simulink model "gm_sampleModel1510_2_sub"  (R2023a)
settings: Solver=VariableStepAuto  StartTime=0.0  StopTime=10.0  RelTol=1e-3
libraries: simulink x3
settings Model: Creator=user1  LastModifiedBy=user1
settings OptimizationCC: BlockReduction=off  ConditionallyExecuteInputs=off
settings DebuggingCC: InheritedTsInSrcMsg=none

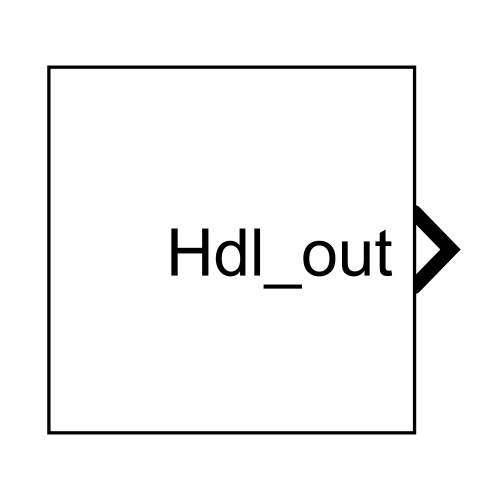
[thumbnail: Simulink's stored preview of the top-level diagram]
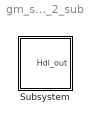
== system gm_sampleModel1510_2_sub ==
  Subsystem : Subsystem

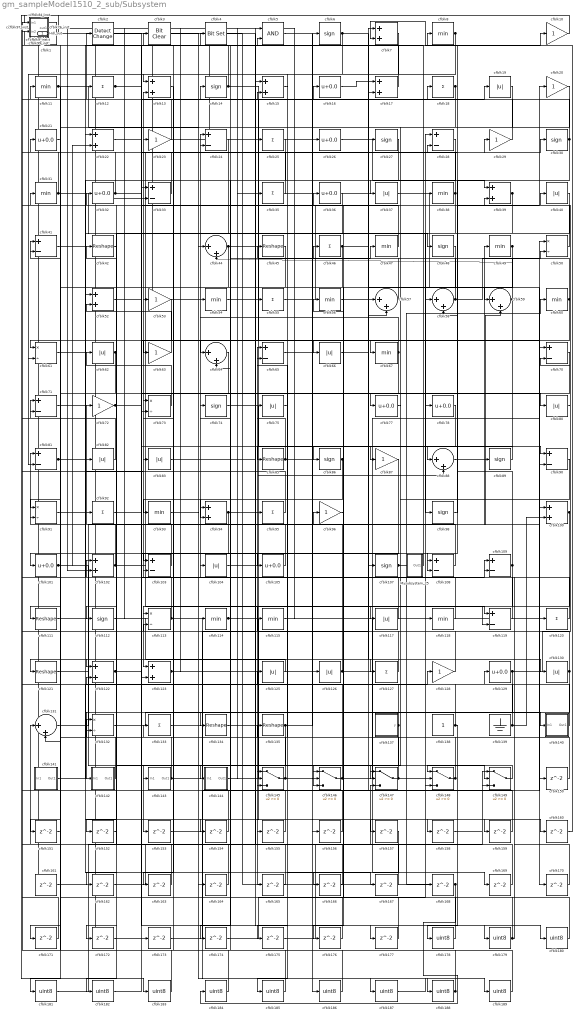
== system gm_sampleModel1510_2_sub/Subsystem ==
  Mysubsystem_25 : Subsystem
  cfblk1 : RelationalOperator  Operator=<=  OutDataTypeStr=boolean  InputSameDT=off
  cfblk{10,20,23,29,53,63,72,87,96,128} (10 alike) : Gain  OutDataTypeStr=uint8
  cfblk{7,13,15,17,22,39,52,94,100,102,122..123} (12 alike) : Sum  OutDataTypeStr=uint8
  cfblk{16,21,26,32,36,77..78,101,105,129} (10 alike) : Bias  Bias=0.0  SaturateOnIntegerOverflow=off
  cfblk{24,28,33,41,65,70..71,81,90,103,108..109,119} (13 alike) : Sum  Inputs=+-  OutDataTypeStr=uint8
  cfblk{19,37,40,62,66,75,80,82..83,104,117,125..126,130} (14 alike) : Abs  OutDataTypeStr=uint8  SaturateOnIntegerOverflow=off
  cfblk106_inst : Subsystem
  cfblk{6,14,27,30,48,74,86,89,98,107,112} (11 alike) : Signum
  cfblk{8,11,31,38,47,49,54,56,60,67,93,114..115,118} (14 alike) : MinMax  OutDataTypeStr=uint8
  cfblk110_inst : Subsystem
  cfblk{42,45,85,111,121,134..135} (7 alike) : Reshape
  cfblk{50,61,73,91,113,132} (6 alike) : Product  Inputs=*/  OutDataTypeStr=uint8  RndMeth=Zero  SaturateOnIntegerOverflow=on
  cfblk116_inst : Subsystem
  cfblk{12,18,25,35,46,55,92,95,120,127,133} (11 alike) : Sum  Inputs=+  OutDataTypeStr=uint8
  cfblk124_inst : Subsystem
  cfblk{44,57..59,64,88,131} (7 alike) : Sum  Inputs=|++  OutDataTypeStr=uint8
  cfblk137 : Subsystem  mask(Counter Free-Running){NumBits=double(16), tsamp=double(-1)}
      mask prompts: NumBits "Simulink:masks:NumberOfBits_MP"; tsamp "Simulink:masks:SampleTime_MP"
      mask help: Simulink:masks:CounterFreeRunning_MD
  cfblk138 : Constant  OutDataTypeStr=uint8  SampleTime=-1
  cfblk139 : Ground
  cfblk140 : Subsystem
  cfblk141 : Subsystem
  cfblk142 : Subsystem
  cfblk143 : Subsystem
  cfblk144 : Subsystem
  cfblk{145..149} (5 alike) : Switch  OutDataTypeStr=uint8  SaturateOnIntegerOverflow=off  InputSameDT=off
  cfblk{150..177} (28 alike) : Delay  SampleTime=1
  cfblk{178..189} (12 alike) : DataTypeConversion  OutDataTypeStr=uint8  SaturateOnIntegerOverflow=off  RndMeth=Floor
  cfblk2 : simulink/Logic and Bit Operations/Detect Change  vinit=0  OutDataTypeStr=uint8
      settings: LibrarySourceBlock=|
      | hdlsllib/Logic and Bit
      | Operations/Detect
      | Change
  cfblk3 : simulink/Logic and Bit Operations/Bit Clear  iBit=0
      settings: LibrarySourceBlock=|
      | hdlsllib/Logic and Bit
      | Operations/Bit Clear
  cfblk34_inst : Subsystem
  cfblk4 : simulink/Logic and Bit Operations/Bit Set  iBit=0
      settings: LibrarySourceBlock=|
      | hdlsllib/Logic and Bit
      | Operations/Bit Set
  cfblk43_inst : Subsystem
  cfblk5 : Logic  AllPortsSameDT=off  OutDataTypeStr=boolean
  cfblk51_inst : Subsystem
  cfblk68_inst : Subsystem
  cfblk69_inst : Subsystem
  cfblk76_inst : Subsystem
  cfblk84_inst : Subsystem
  cfblk97_inst : Subsystem
  cfblk99_inst : Subsystem
  cfblk9_inst : Subsystem
  Hdl_out : Outport  OutDataTypeStr=uint8  SampleTime=1
  wires:
  Mysubsystem_25/1(Out1) -> cfblk51_inst/2(in2)
  cfblk1/1 -> cfblk183/1
  cfblk10/1 -> cfblk69_inst/1(in1)
  cfblk100/1 -> cfblk24/1, cfblk123/1
  cfblk101/1 -> cfblk22/2, cfblk149/2
  cfblk102/1 -> cfblk119/1, cfblk72/1, cfblk29/1
  cfblk103/1 -> cfblk81/1
  cfblk104/1 -> cfblk30/1
  cfblk105/1 -> cfblk92/1
  cfblk106_inst/1(out1) -> cfblk118/1
  cfblk107/1 -> cfblk168/1, cfblk60/1
  cfblk108/1 -> cfblk42/1
  cfblk109/1 -> cfblk14/1, cfblk165/1
  cfblk11/1 -> cfblk44/1, cfblk111/1
  cfblk110_inst/1(out1) -> cfblk126/1
  cfblk111/1 -> cfblk50/1
  cfblk112/1 -> cfblk156/1
  cfblk113/1 -> cfblk68_inst/1(in1), cfblk52/2, cfblk167/1
  cfblk114/1 -> cfblk158/1, cfblk18/1
  cfblk115/1 -> cfblk160/1
  cfblk116_inst/1(out1) -> cfblk26/1, cfblk173/1, cfblk114/1
  cfblk117/1 -> cfblk41/1
  cfblk118/1 -> cfblk52/1
  cfblk119/1 -> cfblk13/2
  cfblk12/1 -> cfblk77/1, cfblk108/2
  cfblk120/1 -> cfblk104/1
  cfblk121/1 -> cfblk59/2
  cfblk122/1 -> cfblk24/2, cfblk109/1
  cfblk123/1 -> cfblk88/2, cfblk47/1
  cfblk124_inst/1(out1) -> cfblk33/2
  cfblk125/1 -> cfblk121/1
  cfblk126/1 -> cfblk53/1, cfblk169/1, cfblk11/1
  cfblk127/1 -> cfblk65/1
  cfblk128/1 -> cfblk115/1
  cfblk129/1 -> cfblk70/2, cfblk142/1(In1)
  cfblk13/1 -> cfblk103/1
  cfblk130/1 -> cfblk145/3, cfblk106_inst/2(in2)
  cfblk131/1 -> cfblk49/1
  cfblk132/1 -> cfblk140/1(In1)
  cfblk133/1 -> cfblk188/1
  cfblk134/1 -> cfblk57/1
  cfblk135/1 -> cfblk6/1, cfblk153/1, cfblk152/1
  cfblk137/1(y) -> cfblk146/3, cfblk73/1
  cfblk138/1 -> cfblk178/1, cfblk23/1
  cfblk139/1 -> cfblk125/1, cfblk100/2
  cfblk14/1 -> cfblk110_inst/1(in1), cfblk170/1
  cfblk140/1(Out1) -> cfblk71/1
  cfblk141/1(Out1) -> cfblk128/1
  cfblk142/1(Out1) -> cfblk106_inst/1(in1)
  cfblk143/1(Out1) -> cfblk146/1, cfblk116_inst/2(in2), cfblk35/1
  cfblk144/1(Out1) -> cfblk17/2
  cfblk145/1 -> cfblk103/2, cfblk159/1
  cfblk146/1 -> cfblk70/1, cfblk62/1, cfblk124_inst/2(in2)
  cfblk147/1 -> cfblk96/1, cfblk144/1(In1)
  cfblk148/1 -> cfblk82/1, cfblk135/1
  cfblk149/1 -> cfblk148/1
  cfblk15/1 -> cfblk145/1
  cfblk150/1 -> cfblk65/2
  cfblk151/1 -> cfblk91/2
  cfblk152/1 -> cfblk102/1
  cfblk153/1 -> cfblk90/2
  cfblk154/1 -> cfblk41/2
  cfblk155/1 -> cfblk97_inst/2(in2)
  cfblk156/1 -> cfblk132/1
  cfblk157/1 -> cfblk185/1
  cfblk158/1 -> cfblk149/3
  cfblk159/1 -> cfblk71/2
  cfblk16/1 -> cfblk17/1
  cfblk160/1 -> cfblk7/2
  cfblk161/1 -> cfblk28/1
  cfblk162/1 -> cfblk149/1
  cfblk163/1 -> cfblk69_inst/2(in2)
  cfblk164/1 -> cfblk99_inst/2(in2)
  cfblk165/1 -> cfblk122/2
  cfblk166/1 -> cfblk131/1
  cfblk167/1 -> cfblk147/3
  cfblk168/1 -> cfblk184/1, Hdl_out/1
  cfblk169/1 -> cfblk110_inst/2(in2)
  cfblk17/1 -> cfblk43_inst/1(in1)
  cfblk170/1 -> cfblk109/2
  cfblk171/1 -> cfblk34_inst/2(in2)
  cfblk172/1 -> cfblk39/2
  cfblk173/1 -> cfblk57/2
  cfblk174/1 -> cfblk148/3
  cfblk175/1 -> cfblk58/1
  cfblk176/1 -> cfblk64/2
  cfblk177/1 -> cfblk31/1
  cfblk178/1 -> cfblk4/1
  cfblk179/1 -> cfblk129/1, cfblk113/2
  cfblk18/1 -> cfblk15/2, cfblk67/1
  cfblk180/1 -> cfblk36/1
  cfblk181/1 -> cfblk5/1
  cfblk182/1 -> cfblk5/2
  cfblk183/1 -> cfblk21/1
  cfblk184/1 -> cfblk1/1
  cfblk185/1 -> cfblk1/2
  cfblk186/1 -> cfblk3/1
  cfblk187/1 -> cfblk189/1
  cfblk188/1 -> cfblk97_inst/1(in1), cfblk9_inst/2(in2), cfblk74/1
  cfblk189/1 -> cfblk133/1
  cfblk19/1 -> cfblk147/2
  cfblk2/1 -> cfblk90/1
  cfblk20/1 -> cfblk151/1
  cfblk21/1 -> cfblk91/1
  cfblk22/1 -> cfblk19/1
  cfblk23/1 -> cfblk9_inst/1(in1)
  cfblk24/1 -> cfblk63/1
  cfblk25/1 -> cfblk134/1
  cfblk26/1 -> cfblk39/1
  cfblk27/1 -> cfblk132/2
  cfblk28/1 -> cfblk37/1
  cfblk29/1 -> cfblk2/1
  cfblk3/1 -> cfblk187/1
  cfblk30/1 -> cfblk88/1, cfblk84_inst/1(in1)
  cfblk31/1 -> cfblk78/1, cfblk76_inst/2(in2)
  cfblk32/1 -> cfblk66/1, cfblk124_inst/1(in1)
  cfblk33/1 -> cfblk76_inst/1(in1)
  cfblk34_inst/1(out1) -> cfblk12/1
  cfblk35/1 -> cfblk116_inst/1(in1)
  cfblk36/1 -> cfblk162/1
  cfblk37/1 -> cfblk100/1
  cfblk38/1 -> cfblk64/1, cfblk15/1
  cfblk39/1 -> cfblk146/2, cfblk93/1
  cfblk4/1 -> cfblk179/1
  cfblk40/1 -> cfblk145/2
  cfblk41/1 -> cfblk48/1
  cfblk42/1 -> cfblk182/1
  cfblk43_inst/1(out1) -> cfblk161/1
  cfblk44/1 -> cfblk94/2, cfblk123/2, cfblk107/1
  cfblk45/1 -> cfblk94/1
  cfblk46/1 -> cfblk73/2, cfblk10/1
  cfblk47/1 -> cfblk68_inst/2(in2)
  cfblk48/1 -> cfblk101/1
  cfblk49/1 -> cfblk58/2, cfblk176/1
  cfblk5/1 -> cfblk180/1
  cfblk50/1 -> cfblk8/1
  cfblk51_inst/1(out1) -> cfblk38/1
  cfblk52/1 -> cfblk80/1
  cfblk53/1 -> cfblk61/1
  cfblk54/1 -> cfblk98/1
  cfblk55/1 -> cfblk20/1
  cfblk56/1 -> cfblk59/1
  cfblk57/1 -> cfblk51_inst/1(in1)
  cfblk58/1 -> cfblk50/2, cfblk46/1
  cfblk59/1 -> cfblk86/1, cfblk45/1, cfblk44/2
  cfblk6/1 -> cfblk13/1, cfblk119/2
  cfblk60/1 -> cfblk84_inst/2(in2), cfblk108/1, cfblk113/1
  cfblk61/1 -> cfblk166/1
  cfblk62/1 -> cfblk122/1, cfblk171/1
  cfblk63/1 -> cfblk32/1
  cfblk64/1 -> cfblk131/2
  cfblk65/1 -> cfblk186/1
  cfblk66/1 -> cfblk130/1
  cfblk67/1 -> cfblk163/1, cfblk54/1
  cfblk68_inst/1(out1) -> cfblk120/1
  cfblk69_inst/1(out1) -> cfblk27/1
  cfblk7/1 -> cfblk85/1
  cfblk70/1 -> cfblk172/1
  cfblk71/1 -> cfblk7/1
  cfblk72/1 -> cfblk33/1, cfblk16/1
  cfblk73/1 -> cfblk22/1
  cfblk74/1 -> cfblk150/1
  cfblk75/1 -> cfblk175/1
  cfblk76_inst/1(out1) -> cfblk141/1(In1)
  cfblk77/1 -> cfblk147/1
  cfblk78/1 -> cfblk105/1
  cfblk8/1 -> cfblk81/2, cfblk61/2
  cfblk80/1 -> cfblk40/1
  cfblk81/1 -> cfblk155/1, cfblk154/1
  cfblk82/1 -> cfblk34_inst/1(in1)
  cfblk83/1 -> cfblk95/1
  cfblk84_inst/1(out1) -> cfblk43_inst/2(in2)
  cfblk85/1 -> cfblk75/1, cfblk127/1
  cfblk86/1 -> cfblk174/1, cfblk143/1(In1)
  cfblk87/1 -> cfblk181/1
  cfblk88/1 -> cfblk89/1
  cfblk89/1 -> cfblk87/1
  cfblk9_inst/1(out1) -> cfblk55/1
  cfblk90/1 -> cfblk117/1
  cfblk91/1 -> cfblk83/1
  cfblk92/1 -> cfblk177/1
  cfblk93/1 -> cfblk164/1
  cfblk94/1 -> cfblk112/1, cfblk157/1
  cfblk95/1 -> cfblk99_inst/1(in1)
  cfblk96/1 -> cfblk56/1
  cfblk97_inst/1(out1) -> cfblk148/2, cfblk102/2
  cfblk98/1 -> cfblk28/2
  cfblk99_inst/1(out1) -> cfblk25/1

== system gm_sampleModel1510_2_sub/Subsystem/Mysubsystem_25 ==
  cfblk136 : Ground
  cfblk79 : Reshape
  Out1 : Outport  SampleTime=1
  wires:
  cfblk136/1 -> cfblk79/1
  cfblk79/1 -> Out1/1

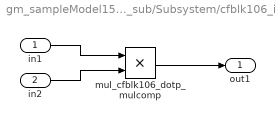
== system gm_sampleModel1510_2_sub/Subsystem/cfblk106_inst ==
  in1 : Inport  OutDataTypeStr=uint8  SampleTime=1
  in2 : Inport  Port=2  OutDataTypeStr=uint8  SampleTime=1
  mul_cfblk106_dotp_mulcomp : Product  Inputs=**  OutDataTypeStr=uint8  SampleTime=1
  out1 : Outport  OutDataTypeStr=uint8  SampleTime=1
  wires:
  in1/1 -> mul_cfblk106_dotp_mulcomp/1
  in2/1 -> mul_cfblk106_dotp_mulcomp/2
  mul_cfblk106_dotp_mulcomp/1 -> out1/1

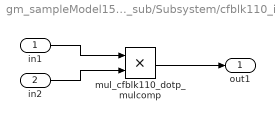
== system gm_sampleModel1510_2_sub/Subsystem/cfblk110_inst ==
  in1 : Inport  OutDataTypeStr=uint8  SampleTime=1
  in2 : Inport  Port=2  OutDataTypeStr=uint8  SampleTime=1
  mul_cfblk110_dotp_mulcomp : Product  Inputs=**  OutDataTypeStr=uint8  SampleTime=1
  out1 : Outport  OutDataTypeStr=uint8  SampleTime=1
  wires:
  in1/1 -> mul_cfblk110_dotp_mulcomp/1
  in2/1 -> mul_cfblk110_dotp_mulcomp/2
  mul_cfblk110_dotp_mulcomp/1 -> out1/1

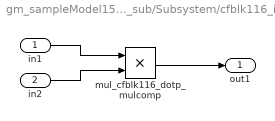
== system gm_sampleModel1510_2_sub/Subsystem/cfblk116_inst ==
  in1 : Inport  OutDataTypeStr=uint8  SampleTime=1
  in2 : Inport  Port=2  OutDataTypeStr=uint8  SampleTime=1
  mul_cfblk116_dotp_mulcomp : Product  Inputs=**  OutDataTypeStr=uint8  SampleTime=1
  out1 : Outport  OutDataTypeStr=uint8  SampleTime=1
  wires:
  in1/1 -> mul_cfblk116_dotp_mulcomp/1
  in2/1 -> mul_cfblk116_dotp_mulcomp/2
  mul_cfblk116_dotp_mulcomp/1 -> out1/1

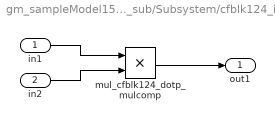
== system gm_sampleModel1510_2_sub/Subsystem/cfblk124_inst ==
  in1 : Inport  OutDataTypeStr=uint8  SampleTime=1
  in2 : Inport  Port=2  OutDataTypeStr=uint8  SampleTime=1
  mul_cfblk124_dotp_mulcomp : Product  Inputs=**  OutDataTypeStr=uint8  SampleTime=1
  out1 : Outport  OutDataTypeStr=uint8  SampleTime=1
  wires:
  in1/1 -> mul_cfblk124_dotp_mulcomp/1
  in2/1 -> mul_cfblk124_dotp_mulcomp/2
  mul_cfblk124_dotp_mulcomp/1 -> out1/1

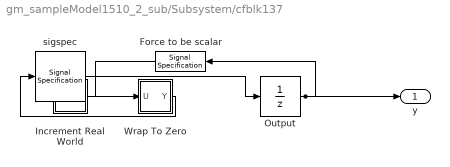
== system gm_sampleModel1510_2_sub/Subsystem/cfblk137 ==
  Force to be scalar : SignalSpecification  DisableCoverage=on  Dimensions=1
  Increment Real World : Subsystem  mask(Real World Value Increment){}
      mask help: Simulink:masks:RealWorldValueIncrement_MD
      mask Display: disp('V++')
  Output : UnitDelay  InitialCondition=0.0  SampleTime=tsamp  HasFrameUpgradeWarning=on
  Wrap To Zero : Subsystem  mask(Wrap To Zero){Threshold=double(65535)}
      mask prompts: Threshold "Simulink:masks:Threshold_MP"
      mask help: Simulink:masks:WrapToZero_MD
  sigspec : SignalSpecification  OutDataTypeStr=uint16  Dimensions=1
  y : Outport  SampleTime=1
  wires:
  Force to be scalar/1 -> Increment Real World/1(u)
  Increment Real World/1(y) -> Wrap To Zero/1(U)
  Output/1 -> Force to be scalar/1, y/1
  Wrap To Zero/1(Y) -> sigspec/1
  sigspec/1 -> Output/1

== system gm_sampleModel1510_2_sub/Subsystem/cfblk140 ==
  In1 : Inport  OutDataTypeStr=uint8  PortDimensions=1  SampleTime=1
  Out1 : Outport  SampleTime=1
  wires:
  In1/1 -> Out1/1

== system gm_sampleModel1510_2_sub/Subsystem/cfblk141 ==
  In1 : Inport  OutDataTypeStr=uint8  PortDimensions=1  SampleTime=1
  Out1 : Outport  SampleTime=1
  wires:
  In1/1 -> Out1/1

== system gm_sampleModel1510_2_sub/Subsystem/cfblk142 ==
  In1 : Inport  OutDataTypeStr=uint8  PortDimensions=1  SampleTime=1
  Out1 : Outport  SampleTime=1
  wires:
  In1/1 -> Out1/1

== system gm_sampleModel1510_2_sub/Subsystem/cfblk143 ==
  In1 : Inport  OutDataTypeStr=uint8  PortDimensions=1  SampleTime=1
  Out1 : Outport  SampleTime=1
  wires:
  In1/1 -> Out1/1

== system gm_sampleModel1510_2_sub/Subsystem/cfblk144 ==
  In1 : Inport  OutDataTypeStr=uint8  PortDimensions=1  SampleTime=1
  Out1 : Outport  SampleTime=1
  wires:
  In1/1 -> Out1/1

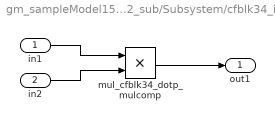
== system gm_sampleModel1510_2_sub/Subsystem/cfblk34_inst ==
  in1 : Inport  OutDataTypeStr=uint8  SampleTime=1
  in2 : Inport  Port=2  OutDataTypeStr=uint8  SampleTime=1
  mul_cfblk34_dotp_mulcomp : Product  Inputs=**  OutDataTypeStr=uint8  SampleTime=1
  out1 : Outport  OutDataTypeStr=uint8  SampleTime=1
  wires:
  in1/1 -> mul_cfblk34_dotp_mulcomp/1
  in2/1 -> mul_cfblk34_dotp_mulcomp/2
  mul_cfblk34_dotp_mulcomp/1 -> out1/1

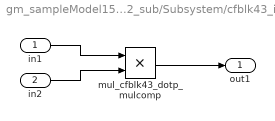
== system gm_sampleModel1510_2_sub/Subsystem/cfblk43_inst ==
  in1 : Inport  OutDataTypeStr=uint8  SampleTime=1
  in2 : Inport  Port=2  OutDataTypeStr=uint8  SampleTime=1
  mul_cfblk43_dotp_mulcomp : Product  Inputs=**  OutDataTypeStr=uint8  SampleTime=1
  out1 : Outport  OutDataTypeStr=uint8  SampleTime=1
  wires:
  in1/1 -> mul_cfblk43_dotp_mulcomp/1
  in2/1 -> mul_cfblk43_dotp_mulcomp/2
  mul_cfblk43_dotp_mulcomp/1 -> out1/1

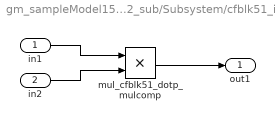
== system gm_sampleModel1510_2_sub/Subsystem/cfblk51_inst ==
  in1 : Inport  OutDataTypeStr=uint8  SampleTime=1
  in2 : Inport  Port=2  OutDataTypeStr=uint8  SampleTime=1
  mul_cfblk51_dotp_mulcomp : Product  Inputs=**  OutDataTypeStr=uint8  SampleTime=1
  out1 : Outport  OutDataTypeStr=uint8  SampleTime=1
  wires:
  in1/1 -> mul_cfblk51_dotp_mulcomp/1
  in2/1 -> mul_cfblk51_dotp_mulcomp/2
  mul_cfblk51_dotp_mulcomp/1 -> out1/1

== system gm_sampleModel1510_2_sub/Subsystem/cfblk68_inst ==
  in1 : Inport  OutDataTypeStr=uint8  SampleTime=1
  in2 : Inport  Port=2  OutDataTypeStr=uint8  SampleTime=1
  mul_cfblk68_dotp_mulcomp : Product  Inputs=**  OutDataTypeStr=uint8  SampleTime=1
  out1 : Outport  OutDataTypeStr=uint8  SampleTime=1
  wires:
  in1/1 -> mul_cfblk68_dotp_mulcomp/1
  in2/1 -> mul_cfblk68_dotp_mulcomp/2
  mul_cfblk68_dotp_mulcomp/1 -> out1/1

== system gm_sampleModel1510_2_sub/Subsystem/cfblk69_inst ==
  in1 : Inport  OutDataTypeStr=uint8  SampleTime=1
  in2 : Inport  Port=2  OutDataTypeStr=uint8  SampleTime=1
  mul_cfblk69_dotp_mulcomp : Product  Inputs=**  OutDataTypeStr=uint8  SampleTime=1
  out1 : Outport  OutDataTypeStr=uint8  SampleTime=1
  wires:
  in1/1 -> mul_cfblk69_dotp_mulcomp/1
  in2/1 -> mul_cfblk69_dotp_mulcomp/2
  mul_cfblk69_dotp_mulcomp/1 -> out1/1

== system gm_sampleModel1510_2_sub/Subsystem/cfblk76_inst ==
  in1 : Inport  OutDataTypeStr=uint8  SampleTime=1
  in2 : Inport  Port=2  OutDataTypeStr=uint8  SampleTime=1
  mul_cfblk76_dotp_mulcomp : Product  Inputs=**  OutDataTypeStr=uint8  SampleTime=1
  out1 : Outport  OutDataTypeStr=uint8  SampleTime=1
  wires:
  in1/1 -> mul_cfblk76_dotp_mulcomp/1
  in2/1 -> mul_cfblk76_dotp_mulcomp/2
  mul_cfblk76_dotp_mulcomp/1 -> out1/1

== system gm_sampleModel1510_2_sub/Subsystem/cfblk84_inst ==
  in1 : Inport  OutDataTypeStr=uint8  SampleTime=1
  in2 : Inport  Port=2  OutDataTypeStr=uint8  SampleTime=1
  mul_cfblk84_dotp_mulcomp : Product  Inputs=**  OutDataTypeStr=uint8  SampleTime=1
  out1 : Outport  OutDataTypeStr=uint8  SampleTime=1
  wires:
  in1/1 -> mul_cfblk84_dotp_mulcomp/1
  in2/1 -> mul_cfblk84_dotp_mulcomp/2
  mul_cfblk84_dotp_mulcomp/1 -> out1/1

== system gm_sampleModel1510_2_sub/Subsystem/cfblk97_inst ==
  in1 : Inport  OutDataTypeStr=uint8  SampleTime=1
  in2 : Inport  Port=2  OutDataTypeStr=uint8  SampleTime=1
  mul_cfblk97_dotp_mulcomp : Product  Inputs=**  OutDataTypeStr=uint8  SampleTime=1
  out1 : Outport  OutDataTypeStr=uint8  SampleTime=1
  wires:
  in1/1 -> mul_cfblk97_dotp_mulcomp/1
  in2/1 -> mul_cfblk97_dotp_mulcomp/2
  mul_cfblk97_dotp_mulcomp/1 -> out1/1

== system gm_sampleModel1510_2_sub/Subsystem/cfblk99_inst ==
  in1 : Inport  OutDataTypeStr=uint8  SampleTime=1
  in2 : Inport  Port=2  OutDataTypeStr=uint8  SampleTime=1
  mul_cfblk99_dotp_mulcomp : Product  Inputs=**  OutDataTypeStr=uint8  SampleTime=1
  out1 : Outport  OutDataTypeStr=uint8  SampleTime=1
  wires:
  in1/1 -> mul_cfblk99_dotp_mulcomp/1
  in2/1 -> mul_cfblk99_dotp_mulcomp/2
  mul_cfblk99_dotp_mulcomp/1 -> out1/1

== system gm_sampleModel1510_2_sub/Subsystem/cfblk9_inst ==
  in1 : Inport  OutDataTypeStr=uint8  SampleTime=1
  in2 : Inport  Port=2  OutDataTypeStr=uint8  SampleTime=1
  mul_cfblk9_dotp_mulcomp : Product  Inputs=**  OutDataTypeStr=uint8  SampleTime=1
  out1 : Outport  OutDataTypeStr=uint8  SampleTime=1
  wires:
  in1/1 -> mul_cfblk9_dotp_mulcomp/1
  in2/1 -> mul_cfblk9_dotp_mulcomp/2
  mul_cfblk9_dotp_mulcomp/1 -> out1/1

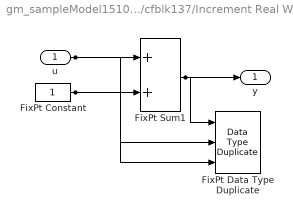
== system gm_sampleModel1510_2_sub/Subsystem/cfblk137/Increment Real World ==
  u : Inport  OutDataTypeStr=uint16  SampleTime=1
  FixPt Constant : Constant  DisableCoverage=on  OutDataTypeStr=Inherit: Inherit via back propagation  SampleTime=-1
  FixPt Data Type Duplicate : DataTypeDuplicate  DisableCoverage=on  NumInputPorts=3
  FixPt Sum1 : Sum  InputSameDT=on  OutDataTypeStr=Inherit: Inherit via back propagation  LockScale=on
  y : Outport  SampleTime=1
  wires:
  u/1 -> FixPt Sum1/1, FixPt Data Type Duplicate/2
  FixPt Constant/1 -> FixPt Sum1/2, FixPt Data Type Duplicate/3
  FixPt Sum1/1 -> FixPt Data Type Duplicate/1, y/1

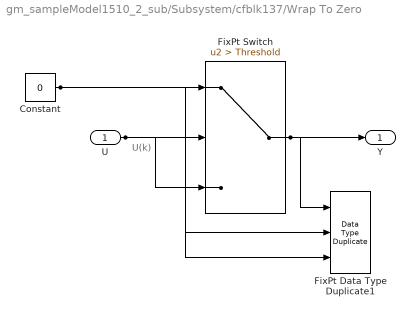
== system gm_sampleModel1510_2_sub/Subsystem/cfblk137/Wrap To Zero ==
  note: U(k)
  U : Inport  OutDataTypeStr=uint16  SampleTime=1
  Constant : Constant  DisableCoverage=on  Value=0  OutDataTypeStr=Inherit: Inherit via back propagation  SampleTime=-1
  FixPt Data Type Duplicate1 : DataTypeDuplicate  DisableCoverage=on  NumInputPorts=3
  FixPt Switch : Switch  Criteria=u2 > Threshold  Threshold=Threshold  OutDataTypeStr=Inherit: Inherit via back propagation  ZeroCross=off  SaturateOnIntegerOverflow=off  InputSameDT=off
  Y : Outport  SampleTime=1
  wires:
  U/1 -> FixPt Switch/3, FixPt Switch/2, FixPt Data Type Duplicate1/2
  Constant/1 -> FixPt Switch/1, FixPt Data Type Duplicate1/3
  FixPt Switch/1 -> FixPt Data Type Duplicate1/1, Y/1
